simulink model "gbyk_v4b (2)"  (R2015a)
settings: Solver=ode4  SolverMode=MultiTasking  StartTime=0.0  StopTime=inf  FixedStep=BKIN_STEP_TIME  RelTol=1e-3
StartFcn:
  |  warndlg('Dexterit-E models cannot run under simulation. Please compile your model and run it from within Dexterit-E.');set_param(bdroot,'SimulationCommand','stop')
model workspace (MAT data in the model file):
  BKIN_STEP_TIME = 0.00025
  col_x = 1
  col_y = 2
  INIT_COLOR = 5
  DELAY_POST_TRIAL = 8
  BKIN_KINEMATIC_FRAME_SIZE = 400
  HIT_COLOR = 6
  E_NO_EVENT = 0
  START_TARGET_COL = 1
  MAX_REACH_TIME_COL = 7
  K_DELAY_FIXED = 3
  K_DELAY_RAND = 4
  K_TRIGGER_VEL = 5
  K_TRIGGER_POS = 6
  K_THRESH_VELMAX = 7
  E_NEW_TRIAL = 1
  E_STAY_START = 2
  E_TARGET_TRIGGER = 5
  E_HIT_TARGET = 10
  E_MISS_TARGET = 11
  K_REWARD_VAL = 1
  VISUAL_RADIUS = 3
  LOGICAL_RADIUS = 4
  STROKE_WIDTH = 7
  TEXT_COLOR = 8
  LABEL_HEIGHT = 10
  E_TOO_SLOW = 20
  K_SCORETEXT_ROW = 2
  LABEL = 9
  E_TARGETS_ON = 3
  DISPLAY_TRIAL_COL = 9
  E_SHOW_INSTRUCT = 25
  E_SHOW_SCORE = 26
  INSTRUCT_PAUSE_BTN = 2
  LABELONLY_X = 11
  LABELONLY_Y = 12
  K_PRE_REWARD_DELAY = 8
  CORR_TGT = 2
  INCORR_TGT = 3
  TGT_C_RWD_FRAC = 6
  BOX_HEIGHT = 13
  B1 = 10
  B2 = 11
  RWD_TARGETC1_COL = 4
  RWD_TARGETC2_COL = 5
undefined symbols (not defined in the file): slselsubs
libraries: Video x7, slrtlib x6, General x3, KINARM_general x3, simulink x1, xpcnilib x1
(part 2 of 2)

== stateflow chart gbyk_v4b (2)/Trial_Control ==
  settings: sampleTime=0.001
  state Initialize/
    // Both the targets and data logging are initially off.
    targetA_state = 0;
    targetB_state[1] = 0;
    targetB_state[2] = 0;
    targetC_state[1] = 0;
    targetC_state[2] = 0;
    targetC_row[1] = 10;
    targetC_row[2] = 11;
    boxState = 0;
    boxRow = 8;
    logging_enable = 0;
    score = 0;
    reward = 0;
    doreward = 0;
    feedback_text = 0;
    repeat_trial_flag = 0;
    setup_trial_flag = false;
  state MainTrial
    state ShowStartTarget/
      // Turn on first target, enable data logging, and wait for a specified time or until the hand is in the target.
      targetA_row = Trial_Protocol[START_TARGET_COL];
      targetA_state = 1;
      logging_enable = 1;
      veltrig = 0;
      postrig = 0;
      disttrig = 0;
      vmaxhit = 0;
      targetB_state[1] = 0;
      targetB_state[2] = 0;
      targetC_state[1] = 0;
      targetC_state[2] = 0;
      boxState = 0;
      tone = 0;
      reward = 0;
    state SetupTgtB/
      //if turning the targets on the for the first time (each trial), set them up. We can only do this once per trial or it will throw the counters off.
      targetB_row[1] = Trial_Protocol[B1];
      targetB_row[2] = Trial_Protocol[B2];
      corrTgt = Trial_Protocol[CORR_TGT] ;
      incorrTgt = Trial_Protocol[INCORR_TGT];
      offeredRewards[1] = Trial_Protocol[RWD_TARGETC1_COL]*Trial_Protocol[TGT_C_RWD_FRAC];
      offeredRewards[2] = Trial_Protocol[RWD_TARGETC2_COL]*Trial_Protocol[TGT_C_RWD_FRAC];
      offeredRewardsC[1] = Trial_Protocol[RWD_TARGETC1_COL];
      offeredRewardsC[2] = Trial_Protocol[RWD_TARGETC2_COL];
      setup_trial_flag = true;
    state StayAtFirstTarget/
      // Log an event that target was reached and wait for a specified time.
      // The wait time may have both a fixed and a random component. The hand must stay in the target for the full wait time.
      event_code = E_STAY_START;
      targetA_state = 1;
      tickCount = TaskwideParams[K_PRE_REWARD_DELAY];
      //TODO ask aaron if we want to show the second row values too or show nothing or just what to show before the trial starts
    state ShowAllTargets/
      // Log an event that target was reached and wait for a specified time.
      // The wait time may have both a fixed and a random component. The hand must stay in the target for the full wait time.
      event_code = E_STAY_START;
      //targetA_state = 1;
      tickCount = TaskwideParams[K_DELAY_FIXED] + TaskwideParams[K_DELAY_RAND] * rand() / RAND_MAX;
      //Show targets before the go tone - allows for comparison
      targetB_state[1] = 1;
      targetB_state[2] = 1;
      targetC_state[1] = 1;
      targetC_state[2] = 1;
      boxState = 1;
    state ShowReachTargets/
      // Turn on all reach targets and log an event indicating this has occurred. Then wait until the hand is the target or until a specified time has elapsed.
      event_code = E_TARGETS_ON;
      tickCount = Trial_Protocol[MAX_REACH_TIME_COL];
      tone = 1;
      during:
      //handvel2d = sqrt((HandVel[1])^2 + (HandVel[2])^2);
      veltrig =  (HandVel > TaskwideParams[K_TRIGGER_VEL]);
      postrig = abs(HandTgtDistance[targetA_row]) > TaskwideParams[K_TRIGGER_POS]; //TODO change this to be !box trig
      boxtrig = HandInBox[boxRow] == 1;
    state TriggerTargetC/
      // TODO event_code = E_BOX_TRIGGER;
      targetB_state[1] = 0;
      targetB_state[2] = 0;
      tone = 0;
    state TriggerTargetB/
      // if they have chosen to go for the box
      //event_code = E_CHOSE_ROW_B
      targetC_state[1] = 0;
      targetC_state[2] = 0;
      boxState = 0;
      tone = 0
      tgtdist = ( (TargetTable[targetB_row[corrTgt]][col_x] - TargetTable[targetA_row][col_x])^2.0 + (TargetTable[targetB_row[corrTgt]][col_y] - TargetTable[targetA_row][col_y])^2.0 )^0.5;
      during:
      postrig = HandInTarget[targetB_row[corrTgt]]==1;
      tgt2trig = HandInTarget[targetB_row[incorrTgt]] ==1;
      disttrigy = (HandPos[2]) > (TargetTable[targetB_row[corrTgt]][col_y])*0.01;
      disttrig = abs(HandTgtDistance[targetA_row]) > (tgtdist)*0.01;
      disttrig = disttrig && ( (TargetTable[targetB_row[corrTgt]][col_y] != TargetTable[targetA_row][col_y]) && disttrigy);
      vmaxhit = (vmaxhit || (HandVel > TaskwideParams[K_THRESH_VELMAX]));  //(sqrt(HandVel[1]^2 + HandVel[2]^2)
    state RevealCorrectTgtC/
      //event_code = E_CHOSE_TGT_C
      targetC_state[corrTgt] = 1;
      targetC_state[incorrTgt] = 0;
      during:
      //TODO fix this below
      disttrigy = (HandPos[2]) > (TargetTable[targetC_row[corrTgt]][col_y])+1;
      disttrig = abs(HandTgtDistance[targetA_row]) > (tgtdist)*0.01;
      disttrig = disttrig && disttrigy;
      postrig = HandInTarget[targetC_row[corrTgt]] ==1;
      vmaxhit = (vmaxhit || (HandVel > TaskwideParams[K_THRESH_VELMAX]));
    state TooSlowC/
      // Log a bad trial
      //event_code = E_TOO_SLOW;
      targetC_state[1] = 0;
      targetC_state[2] = 0;
      boxState = 0;
      repeat_trial_flag = 1;
      reward = 0;
      doreward = 0;
      feedback_text = -1;
      tone = 2
      tickCount = 500;
    state HitTargetC/
      // Log a successful hit
      //event_code = E_HIT_TARGETC;
      targetC_state[corrTgt] = 3;
      targetC_state[incorrTgt] = 0;
      doreward = 1;
      reward = offeredRewardsC[1];
      score += reward;
      tone = 3;
      boxState = 0
      tickCount = 500;
    state MissTargetC/
      // Log a target miss
      //event_code = E_MISS_TARGETC;
      targetC_state[1] = 0;
      targetC_state[2] = 0;
      boxState =0;
      tone = 2;
      reward = 0;
      doreward = 0;
      tickCount = 500;
    state HitTargetB/
      // Log a successful hit
      //event_code = E_HIT_TARGETB;
      targetB_state[corrTgt] = 3;
      targetB_state[incorrTgt] = 0;
      doreward = 1;
      reward = offeredRewards[1];
      score += reward;
      tone = 3;
      tickCount = 500;
    state MissTargetB/
      // Log a target miss
      //event_code = E_MISS_TARGETB;
      targetB_state[1] = 0;
      targetB_state[2] = 0;
      reward = 0;
      doreward = 0;
      tone = 2;
      tickCount = 500;
    state TooSlow/
      // Log a bad trial
      event_code = E_TOO_SLOW;
      targetB_state[1] = 0;
      targetB_state[2] = 0;
      targetC_state[1] = 0;
      targetC_state[2] = 0;
      boxState = 0;
      repeat_trial_flag = 1;
      reward = 0;
      doreward = 0;
      feedback_text = -1;
      tone = 2
      tickCount = 500;
    state EndOfTrial/
      // Set the post-trial delay.
      tickCount = Trial_Protocol[DELAY_POST_TRIAL];
    StayAtFirstTarget -> ShowStartTarget [order 2] : [HandInTarget[targetA_row] == 0]
    ShowStartTarget -> (junction 139)
    (junction 139) -> SetupTgtB [order 1] : [HandInTarget[targetA_row] == 1 && !setup_trial_flag]
    (junction 139) -> StayAtFirstTarget [order 2] : [HandInTarget[targetA_row] == 1 && setup_trial_flag]
    SetupTgtB -> StayAtFirstTarget
    StayAtFirstTarget -> ShowAllTargets [order 1] : after(tickCount, e_clk)
    ShowAllTargets -> ShowReachTargets : after(tickCount,e_clk)
    ShowReachTargets -> TooSlow [order 1] : after(tickCount, e_clk)/
        | feedback_text = -2;
        | //if the trial times out it is an error
    ShowReachTargets -> TriggerTargetC [order 3] : [after(1,e_clk) && veltrig && boxtrig]
    ShowReachTargets -> TriggerTargetB [order 2] : [after(1,e_clk) && veltrig && postrig && !boxtrig]
        | //when the hand velocity pr position exceeds the threshold
        | //shut off the second target
    TriggerTargetC -> RevealCorrectTgtC : after(1,e_clk)
    RevealCorrectTgtC -> TooSlowC [order 1] : [(after(1,e_clk) && (disttrig || postrig) && vmaxhit == 0) || after(tickCount, e_clk)]
        | //check if missed the target but moved fast enough
    RevealCorrectTgtC -> MissTargetC [order 3] : [after(1,e_clk) && (disttrig && !postrig) && vmaxhit]/
        | //check if missed the target but moved fast enough
    RevealCorrectTgtC -> HitTargetC [order 2] : [after(1,e_clk) && postrig && vmaxhit]
        | //check if hit the target and moved fast enough
    TriggerTargetB -> HitTargetB [order 3] : [after(1,e_clk) && postrig && vmaxhit]
        | //check if hit the target and moved fast enough
    TriggerTargetB -> MissTargetB [order 2] : [after(1,e_clk) && (tgt2trig || (disttrig && !postrig)) && vmaxhit]/
        | //check if missed the target but moved fast enough
    TriggerTargetB -> TooSlow [order 1] : [(after(1,e_clk) && (disttrig || postrig) && vmaxhit == 0) || after(tickCount, e_clk)]/
        | feedback_text = -1;
        | //check if missed the target but moved fast enough
    TooSlowC -> EndOfTrial
    MissTargetC -> EndOfTrial
    HitTargetC -> EndOfTrial
    HitTargetB -> EndOfTrial : after(tickCount, e_clk)
    MissTargetB -> EndOfTrial : after(tickCount, e_clk)
    TooSlow -> EndOfTrial : after(tickCount, e_clk)
  state EndInstructPause/
    instruct_num = 0;
    tickCount = Trial_Protocol[DELAY_POST_TRIAL];
    logging_enable = 1;
    score = 0;
  state Ending/
    //end the special "show score" state
    //score = 0;
    e_Trial_End;
  state ReturnToStart1/
    targetA_state=1;
    targetB_state[1] = 0;
    targetB_state[2] = 0;
    targetC_state[1] = 0;
    targetC_state[2] = 0;
    boxState = 0;
    feedback_text = 0;
    doreward = 0;
    repeat_trial_flag = 0;
    logging_enable = 1;
    setup_trial_flag = false;
  state InstructWaitState/
    //"pause" here until the button has been clicked
  state ShowScoreState/
    event_code = E_SHOW_SCORE;
    targetA_state = 0;
    targetB_state[1] = 0;
    targetB_state[2] = 0;
    targetC_state[1] = 0;
    targetC_state[2] = 0;
    boxState = 0;
    doreward = 2;
    tickCount = Trial_Protocol[MAX_REACH_TIME_COL];
    logging_enable = 0;
  state ShowInstructState/
    event_code = E_SHOW_INSTRUCT;
    targetA_state = 0;
    targetB_state[1] = 0;
    targetB_state[2] = 0;
    targetC_state[1] = 0;
    targetC_state[2] = 0;
    boxState = 0;
    doreward = 0;
    instruct_num = Trial_Protocol[DISPLAY_TRIAL_COL];
    tickCount = Trial_Protocol[MAX_REACH_TIME_COL];
    logging_enable = 0;
  state Inter_Trial_State/
    // Turn off both targets, turn off data logging, reset the
    // event code, and send the e_Trial_End Stateflow event.
    event_code = 0;
    targetA_state = 1;
    targetB_state[1] = 0;
    targetB_state[2] = 0;
    targetC_state[1] = 0;
    targetC_state[2] = 0;
    boxState = 0;
    offeredRewards[1] = 0;
    offeredRewards[2] = 0;
    feedback_text = 0;
    doreward = 0;
    setup_trial_flag = false;
    e_Trial_End;
  (default) -> Initialize
  Initialize -> ShowStartTarget [order 1] : [Trial_Protocol[DISPLAY_TRIAL_COL] == 0]
  ReturnToStart1 -> ShowStartTarget : after(1, e_clk)/
  Initialize -> ShowInstructState [order 2] : [Trial_Protocol[DISPLAY_TRIAL_COL] > 0]
      | //in case we start with an instruction trial
  Ending -> (junction 91) : after(1,e_clk)
  (junction 91) -> EndInstructPause [order 1] : [Trial_Protocol[DISPLAY_TRIAL_COL] == 0]/
      | //continue if a regular trial comes after!
  (junction 91) -> ShowInstructState [order 2] : //so we can show the score and then show instructions
      | [Trial_Protocol[DISPLAY_TRIAL_COL] > 0]
  EndInstructPause -> ReturnToStart1 : after(tickCount,e_clk)
  InstructWaitState -> Ending : e_cntl_btn/
      | event_code = 22;
  ShowScoreState -> Ending : after(tickCount,e_clk)
  ShowInstructState -> InstructWaitState : after(tickCount,e_clk)
  (junction 86) -> ReturnToStart1 [order 3] : [Trial_Protocol[DISPLAY_TRIAL_COL] == 0]
  (junction 86) -> ShowScoreState [order 1] : [Trial_Protocol[DISPLAY_TRIAL_COL] == -1]
  (junction 86) -> ShowInstructState [order 2] : [Trial_Protocol[DISPLAY_TRIAL_COL] > 0]
  Inter_Trial_State -> (junction 86) : after(1,e_clk)
  MainTrial -> Inter_Trial_State : e_ExitTrialNow/
      | tickCount = 1;
  EndOfTrial -> Inter_Trial_State : after(tickCount,e_clk)
  data: rwd_val function_output double; TgtRwdRatio function_input double; RwdVal function_input double; FixedRwdRatios1 function_input double; FixedRwdRatios2 function_input double; FixedRwdRatios3 function_input double; tIterations function_input double size=[60, 2]; TPindex function_input double; T1 function_output double; Targ1 function_input double; Targ2 function_input double; Targ1Prob function_input double; NTReps function_input double; T2 function_output double; Targ1Rwd function_input double; Targ2Rwd function_input double; RwdT1 function_output double; RwdT2 function_output double; PT1 function_output double; PT2 function_output double; tIter function_output double size=[60, 2]; r function_input double; logging_enable output double size=[2]; Trial_Protocol input double size=50; TaskwideParams input double; TrialReps input double; CurTPindex input; TargetTable input double; HandInTarget input double; event_code output uint16 [0..] =0; postrig output boolean; veltrig output boolean; disttrig output boolean; vmaxhit output boolean; targetA_row output [1..32]; targetA_state output double; targetB_row output double size=[2]; targetB_state output double size=[2]; offeredRewards output double size=2; score output double; tickCount local double; RAND_MAX constant double =32767; HandTgtDistance input double; HandPos input double; HandVel input double; doreward output double; feedback_text output int32; reward output double; instruct_num output double; tone output double; repeat_trial_flag output double; tgtdist local double; trialIterations output double size=[60, 2] =0; targetC_row output double size=[2]; targetC_state output double size=[2]; offeredRewardsC output double size=[2]; boxRow output double size=1; rwdTgts local double size=2; pTgts local double size=2; setup_trial_flag local boolean; disttrigy local boolean; tgt2trig local double; boxState output double size=1; corrTgt local double; incorrTgt local double; boxtrig local double; HandInBox input double
  data targetA_row settings: description=index of the row currently being used in the TargetTable
  events: e_clk input RISING_EDGE_EVENT; e_ExitTrialNow input EITHER_EDGE_EVENT; e_Trial_End output EITHER_EDGE_EVENT; e_cntl_btn input EITHER_EDGE_EVENT
  function rwd_val = CalcRwd(TgtRwdRatio,RwdVal,FixedRwdRatios1,FixedRwdRatios2,FixedRwdRatios3):
    | function rwd_val = CalcRwd(TgtRwdRatio,RwdVal,FixedRwdRatios1,FixedRwdRatios2,FixedRwdRatios3)
    |  
    | if TgtRwdRatio < -2
    |     rwd_val = RwdVal * FixedRwdRatios3;
    | elseif TgtRwdRatio < -1
    |     rwd_val = RwdVal * FixedRwdRatios2;
    | elseif TgtRwdRatio < 0
    |     rwd_val = RwdVal * FixedRwdRatios1;
    | else %(TgtRwdRatio > 0)
    |     rwd_val = abs(TgtRwdRatio) * RwdVal;
    | end
  function [T1,T2,RwdT1,RwdT2,PT1,PT2,tIter] = SetTargB(tIterations,TPindex,Targ1,Targ2,Targ1Prob,NTReps,Targ1Rwd,Targ2Rwd,r):
    | function [T1,T2,RwdT1,RwdT2,PT1,PT2,tIter] = SetTargB(tIterations,TPindex,Targ1,Targ2,Targ1Prob,NTReps,Targ1Rwd,Targ2Rwd,r)
    | 
    | %trialIterations is a matrix where each row corresponds to a T1TargProb, and
    | %each column counts the number of T1 and T2 iterations previously run.
    | 
    | %index the counter based on probability - but this is wrong because we can
    | %  have multiple unique trials with the same probability. So we need to
    | %  index by TP number instead!
    | %
    | % if abs(Targ1Prob - 0.5) < 1e-5
    | %     i1 = 1;
    | % elseif abs(Targ1Prob - 0.6) < 1e-5
    | %     i1 = 2;
    | % elseif abs(Targ1Prob - 0.7) < 1e-5
    | %     i1 = 3;
    | % elseif abs(Targ1Prob - 0.8) < 1e-5
    | %     i1 = 4;
    | % elseif abs(Targ1Prob - 0.9) < 1e-5
    | %     i1 = 5;
    | % elseif abs(Targ1Prob - 0.1) < 1e-5
    | %     i1 = 6;
    | % elseif abs(Targ1Prob - 0.2) < 1e-5
    | %     i1 = 7;
    | % elseif abs(Targ1Prob - 0.3) < 1e-5
    | %     i1 = 8;
    | % elseif abs(Targ1Prob - 0.4) < 1e-5
    | %     i1 = 9;
    | % elseif abs(Targ1Prob - 0.51) < 1e-5
    | %     i1 = 10;    
    | % end
    | % 
    | % Targ1Prob = round(Targ1Prob*10)/10;
    | % if abs(Targ1Prob - 0.5) < 1e-5
    | %     i1 = 1;
    | % elseif abs(Targ1Prob - 0.625) < 1e-5
    | %     i1 = 2;
    | % elseif abs(Targ1Prob - 0.75) < 1e-5
    | %     i1 = 3;
    | % elseif abs(Targ1Prob - 0.875) < 1e-5
    | %     i1 = 4;
    | % elseif abs(Targ1Prob - 0.125) < 1e-5
    | %     i1 = 5;
    | % elseif abs(Targ1Prob - 0.25) < 1e-5
    | %     i1 = 6;
    | % elseif abs(Targ1Prob - 0.375) < 1e-5
    | %     i1 = 7;
    | % elseif abs(Targ1Prob - 1.500) < 1e-5
    | %     Targ1Prob = Targ1Prob-1; %1.5 is a placeholder so we can have 2 copies of the .5 condition
    | %     i1 = 8;
    | % end
    | 
    | i1 = TPindex; %index into the trial-counter array
    | 
    | if abs(Targ1Prob - 1.500) < 1e-5
    |     Targ1Prob = Targ1Prob-1; %1.5 is a placeholder so we can have 2 copies of the .5 condition
    | end
    | Targ1Prob = round(Targ1Prob*1000)/1000; %clean up the probability value
    | 
    | 
    | %generate a random number
    | %if the random number is less than the T1 probability, set T1 to be the correct
    | %target; otherwise set T2 to be the correct target.
    | %if rand <= Targ1Prob
    | if r <= Targ1Prob
    |     tIterations(i1,1) = tIterations(i1,1)+1;
    |     if tIterations(i1,1) > NTReps*Targ1Prob %too many reps, do the other option
    |         tIterations(i1,1) = tIterations(i1,1)-1;
    |         tIterations(i1,2) = tIterations(i1,2)+1;
    |         
    |         T1 = Targ2; %swap T1 and T2
    |         T2 = Targ1;
    |         RwdT1 = Targ2Rwd;
    |         RwdT2 = Targ1Rwd;
    |         PT1 = 1-Targ1Prob;
    |         PT2 = Targ1Prob;
    |         
    |     else %T1 is good, so keep it as T1
    |         T1 = Targ1;
    |         T2 = Targ2;
    |         RwdT1 = Targ1Rwd;
    |         RwdT2 = Targ2Rwd;
    |         PT1 = Targ1Prob;
    |         PT2 = 1-Targ1Prob;
    |         
    |     end
    | else
    |     tIterations(i1,2) = tIterations(i1,2)+1;
    |     if tIterations(i1,2) > NTReps*(1-Targ1Prob) %too many reps, do the other option
    |         tIterations(i1,2) = tIterations(i1,2)-1;
    |         tIterations(i1,1) = tIterations(i1,1)+1;
    |         
    |         T1 = Targ1; %Use T1
    |         T2 = Targ2;
    |         RwdT1 = Targ1Rwd;
    |         RwdT2 = Targ2Rwd;
    |         PT1 = Targ1Prob;
    |         PT2 = 1-Targ1Prob;
    | 
    |     else
    |         
    |         T1 = Targ2; %we should be doing T2, so swap them
    |         T2 = Targ1;
    |         RwdT1 = Targ2Rwd;
    |         RwdT2 = Targ1Rwd;
    |         PT1 = 1-Targ1Prob;
    |         PT2 = Targ1Prob;
    |         
    |     end
    | end
    | 
    | tIter = tIterations; %update the trial counter and output it back to the state machine

== matlab function gbyk_v4b (2)/AddTxt2TgtB ==
  data: VCODE input; VCODE_MOD output; rewards input
function VCODE_MOD  = rwd_tgt(VCODE,rewards)
%#codegen

VCODE_MOD = VCODE;

%rewards = rwd_multipliers*rwd_val;

for a = 1:length(rewards)

    if any(rewards)>0
        jj = 1;
        label = rewards(a);
        
        if (label < 10)
            VCODE_MOD(a, jj + 14) = int32(label+int32('0'));
            
        elseif (label < 100) %score < $1
            n1 = int32(floor(double(label)/10));  %we need to cast score to a double otherwise the arithmetic is wrong!
            n2 = label - n1*10;
        
            VCODE_MOD(a, jj + 14) = int32(n1+int32('0'));
            jj = jj+1;
            VCODE_MOD(a, jj + 14) = int32(n2+int32('0'));
        else %label < 1000
            n1 = int32(floor(double(label)/100));  %we need to cast score to a double otherwise the arithmetic is wrong!
            n2 = label - n1*100;
            n2 = int32(floor(double(n2)/100));  %we need to cast score to a double otherwise the arithmetic is wrong!
            n3 = label - n1*100 - n2*10;
        
            VCODE_MOD(a, jj + 14) = int32(n1+int32('0'));
            jj = jj+1;
            VCODE_MOD(a, jj + 14) = int32(n2+int32('0'));
            jj = jj+1;
            VCODE_MOD(a, jj + 14) = int32(n3+int32('0'));
        end
        VCODE_MOD(a,jj + 1 + 14) = 0; %terminate string
    else
        VCODE_MOD(a,15) = 0; %terminate string
    end
end

== matlab function gbyk_v4b (2)/KINARM_HandInBox/Embedded MATLAB InsideTarget ==
  settings: fimath=|
      | fimath(...
      | 'RoundMode', 'floor',...
      | 'OverflowMode', 'wrap',...
      | 'ProductMode', 'KeepLSB', 'ProductWordLength', 32,...
      | 'SumMode', 'KeepLSB', 'SumWordLength', 32,...
      | 'CastBeforeSum', false)
  data: handpos input size=2; target_type input; attribcol input; num_targets input; intarget output; Target_Table input
function intarget = FIsInsideTarget(handpos, target_type, attribcol, num_targets, Target_Table)
% all dimensions in m, rad
% arguments:
% handpos: x,y positions of center of target
% attribcol: columns in target table specifying target attributes.  
% Specific to Target_Type
%	circle:
%	[X0,Y0,r...,rn] where:
%	X0,Y0 : centre of circle
%	r : logical radius of circle (i.e. radius used to determine 'in' or 'out' of target)
%	rn: logical radius of other targets (e.g. 2nd, 3rd) also specified in target row.
%   Up to 4 targets can be specified in a row
% ellipse:
%	[X0,Y0,a,b,t...,an, bn, tn] where:
%	X0,Y0 : centre of ellipse
%	a,b : major, minor radii of ellipse
%	t : rotation of ellipse in degrees
%	an,bn : major, minor radii of ellipse of other targets (e.g. 2nd, 3rd) also specified in target row
%	tn : rotation of ellipse in degrees of other targets (e.g. 2nd, 3rd) also specified in target row
%   Up to 4 targets can be specified in a row


target_col_x=1;
target_col_y=2;

x=handpos(1);
y=handpos(2);

intarget = zeros(size(Target_Table,1),5);

X0 = Target_Table(:,target_col_x)*0.01;			%Target Table sizes in cm in v1.4
Y0 = Target_Table(:,target_col_y)*0.01;			%Target Table sizes in cm in v1.4

deltax=x-X0;
deltay=y-Y0;

if target_type==1			%circle
	for target=1:num_targets
		r = Target_Table(:,attribcol(target))*0.01;			%Target Table sizes in cm in v1.4
		% simple euclidean distance
		distance2 = deltax.^2 + deltay.^2;					%distance2 is the square of the distance
	    intarget(:,target) = (distance2 <= r.^2);
	end
elseif target_type==2		%ellipse
	for target=1:num_targets
	    a = Target_Table(:,attribcol(target*3-2))*0.01;			%Target Table sizes in cm in v1.4
	    b = Target_Table(:,attribcol(target*3-1))*0.01;			%Target Table sizes in cm in v1.4	
	    t = Target_Table(:,attribcol(target*3))*(pi / 180.0);	%Target Table angles in degrees in v1.4
		sint=sin(t);
		cost=cos(t);
		xrotate=deltax.*cost+deltay.*sint;		%location of x point in ellipse's coordinate frame
		yrotate=-deltax.*sint+deltay.*cost;		%location of y point in ellipse's coordinate frame
		m=yrotate./xrotate;						%slope of line between the (x,y) to (x0,y0) in ellipse's coordinate frame
		y2sq=1./(1./(m.*a).^2+1./b.^2);			%y2sq is y2^2, where y2 is the intersection of the ellipse and the (x,y) to (x0,y0) line
	    intarget(:,target) = (yrotate.^2 <= y2sq);
    end
elseif target_type==3       %rectangle
    for target=1:num_targets
        w = Target_Table(:,attribcol(target*3-2))*0.01;  %width (sizes in cm in v1.4)
        h = Target_Table(:,attribcol(target*3-1))*0.01;  %height (sizes in cm in v1.4)
        
        if attribcol(target*3) > 0
            t = Target_Table(:,attribcol(target*3))*(pi / 180.0);  %angle (angles in degrees in v1.4)
        else
            t = zeros(size(Target_Table, 1), 1);
        end

        sint=sin(t);
        cost=cos(t);

        xrotate=deltax.*cost + deltay.*sint;   %location of x point in rectangle's coordinate frame
        yrotate=-deltax.*sint + deltay.*cost;  %location of y point in rectangle's coordinate frame

        intarget(:,target) = abs(xrotate) <= w/2 & abs(yrotate) <= h/2;
    end
elseif target_type==4       %line
    for target=1:num_targets
        % treat the line like a rectangle of height h and width w
        % determine height (stroke width) in the same fashion as in Show_Target
        if attribcol(target*3-2) == 0                     %0 column index means stroke width of 0
            h = zeros(size(Target_Table, 1), 1);
        elseif attribcol(target*3-2) < 0                  %-ve column index means stroke width of 1mm
            h = ones(size(Target_Table, 1), 1) .* 0.001;
        else
            h = Target_Table(:,attribcol(target*3-2)) * 0.01;  %target table contains width in cm
        end
        
        ex = Target_Table(:,attribcol(target*3-1))*0.01;  %endpoint in x relative to start point (cm)
        ey = Target_Table(:,attribcol(target*3))*0.01;    %endpoint in y relative to start point (cm)
        
        w = sqrt(ex.^2 + ey.^2);                          %width (cm)
        
        % determine the vector from the line's midpoint to the hand position
        handx = deltax - ex/2;
        handy = deltay - ey/2;
        
        t = atan2(ey, ex);                                %calculate angle of the line (rads)
        sint = sin(t);
        cost = cos(t);
        
        xrotate = handx.*cost + handy.*sint;   %location of x point in rectangle's coordinate frame
        yrotate = -handx.*sint + handy.*cost;  %location of y point in rectangle's coordinate frame
 
        intarget(:,target) = abs(xrotate) <= w/2 & abs(yrotate) <= h/2;
    end
elseif target_type==5  % triangle
    for target=1:num_targets
        w = Target_Table(:,attribcol(target*4-3))*0.01;         %length (sizes in cm in v1.4)
        
        % If a height column of 0 is specified, make the triangle equilateral. Otherwise, use the
        % values for height and peak offset from the target table.
        if attribcol(target*4-2) > 0
            h = Target_Table(:,attribcol(target*4-2))*0.01;  %height (sizes in cm in v1.4)
            p = Target_Table(:,attribcol(target*4-1))*0.01;  %peak offset (sizes in cm in v1.4)
        else
            h = w.*sin(pi/3.0);
            p = zeros(size(Target_Table, 1), 1);
        end
        
        if attribcol(target*4) > 0
            t = Target_Table(:,attribcol(target*4))*(pi / 180.0);  %angle (angles in degrees in v1.4)
        else
            t = zeros(size(Target_Table, 1), 1);
        end
        
        sint = sin(t);
        cost = cos(t);
        
        xrotate = deltax.*cost + deltay.*sint;   %location of x point in triangle's coordinate frame
        yrotate = -deltax.*sint + deltay.*cost;  %location of y point in triangle's coordinate frame
        
        % Perform a point-in-triangle test using Barycentric coordinates.
        A = [-w/2 - p/3, -h/3];
        B = [2*p/3, 2*h/3];
        C = [w/2 - p/3, -h/3];
        
        v0 = C - A;
        v1 = B - A;
        v2 = [xrotate, yrotate] - A;

        dot00 = v0(:,1) .* v0(:,1) + v0(:,2) .* v0(:,2);
        dot01 = v0(:,1) .* v1(:,1) + v0(:,2) .* v1(:,2);
        dot02 = v0(:,1) .* v2(:,1) + v0(:,2) .* v2(:,2);
        dot11 = v1(:,1) .* v1(:,1) + v1(:,2) .* v1(:,2);
        dot12 = v1(:,1) .* v2(:,1) + v1(:,2) .* v2(:,2);

        invDenom = 1 ./ (dot00 .* dot11 - dot01 .* dot01);
        u = (dot11 .* dot02 - dot01 .* dot12) .* invDenom;
        v = (dot00 .* dot12 - dot01 .* dot02) .* invDenom;

        intarget(:,target) = (u > 0) & (v > 0) & (u + v < 1);
    end
end

== matlab function gbyk_v4b (2)/Play Sound/Play sound over and over ==
  data: tone input; output output; beep input; errorbeep input; coin input
function output = fcn(tone,beep,errorbeep,coin)
%#codegen

persistent t last_tone_state
if isempty(t), t = 0; end
if isempty(last_tone_state), last_tone_state = 0; end

trigger = last_tone_state ~= tone;
if trigger > 0
    last_tone_state = tone;
end

output = 0;		% default
if t == 0 && trigger > 0
	% start the playing of the sound.
	t = t + 1;
end

if tone == 1
    data = beep;
elseif tone == 2
    data = errorbeep;
elseif tone == 3
    data = coin;
else 
    t = 0;
    data = 0;
end

if t > 0
	output = data(t);
	if t == length(data)
		t = 0;
	else
		t = t + 1;
	end
end

== matlab function gbyk_v4b (2)/MATLAB Function ==
  data: BlockDef input; ListReps output
function ListReps = calcListReps(BlockDef)
%#codegen

BlockDef = nonzeros(BlockDef);
%BlockDef = BlockDef(2:end);

trials = unique(BlockDef);
reps1 = sum(BlockDef == trials(1));
reps2 = sum(BlockDef == trials(2));
reps3 = sum(BlockDef == trials(3));
ListReps = round(mean([reps1,reps2,reps3]));

== matlab function gbyk_v4b (2)/DisplayText/MATLAB Function ==
  data: VCODE input; score_dbl input; VCODE_mod output; fdbk_text input
function VCODE_mod = fcn(VCODE,score_dbl,fdbk_text)


VCODE_mod = VCODE;

score = round(score_dbl);  %for display purposes, round fractional rewards

if (fdbk_text == 0)  %if this is zero, show the score
       
    
    %score is in cents. potentially need to convert to dollars
    
    if (score < 10)
        text1 = 'You earned ';
        text2 = ' cents!';
        
        textout = [text1 int2char(int32(score)) text2];
        
    elseif (score < 100) %score < $1
        text1 = 'You earned ';
        text2 = ' cents!';
        
        n1 = int32(floor(double(score)/10));  %we need to cast score to a double otherwise the arithmetic is wrong!
        n2 = score - n1*10;
        
        textout = [text1 int2char(int32(n1)) int2char(int32(n2)) text2];
        
    else %score > $1, convert to dollars to keep the score readable
        text1 = 'You earned $';
        text2 = '.';
        text3 = '!';
        
        dollars = int32(floor(double(score)/100));
        if (dollars >= 10) %double digit dollar value
            n1d = int32(floor(double(dollars)/10));
            n2d = dollars - n1d*10;
            textdollars = [int2char(int32(n1d)) int2char(int32(n2d))];
        else %single digit
            textdollars = int2char(int32(dollars));
        end
        
        cents = score-dollars*100;
        if (cents < 10)
            textcents = ['0' int2char(int32(cents))];
        else
            n1 = int32(floor(double(cents)/10));
            n2 = round(cents - n1*10);
            textcents = [int2char(int32(n1)) int2char(int32(n2))];
        end
        
        textout = [text1 textdollars text2 textcents text3];
        
    end
    
elseif (fdbk_text == 1) 
    %print "too fast"
    textout = 'Too Fast!';
    
    
elseif (fdbk_text == 2) 
    %print "too fast"
    textout = 'Too Early!';

elseif (fdbk_text == -1) 
    %print "too slow"
    
    textout = 'Too Slow!';

elseif (fdbk_text == -2) 
    %print "too fast"
    textout = 'Too Late!';


else
    textout = '';
    
end
    

%the first character is VCODE(15)
%need to translate text into ascii:
textnum = double(textout); %this quickly casts each char into a number

%make sure we won't overflow the VCODE: no more than 50 chars! we will
%clip off anything that overflows.
VCODE_mod(1,15:min([15+length(textout),64])) = textnum(1:min([length(textnum),50])); %write out as many the characters as possible into the VCODE
VCODE_mod(1,min([15+length(textout)+1,64])) = 0;  %terminate the string!



function s = int2char(n)

n = mod(n,10); %make sure we only have 1 digit or we will get a weird character!

s = char(n+int32('0')); %// add the character

== matlab function gbyk_v4b (2)/AddTxt2TgtC ==
  data: VCODE input; VCODE_MOD output; rewards input
function VCODE_MOD  = rwd_tgt(VCODE,rewards)
%#codegen

VCODE_MOD = VCODE;

%rewards = rwd_multipliers*rwd_val;

for a = 1:length(rewards)

    if any(rewards)>0
        jj = 1;
        label = rewards(a);
        
        if (label < 10)
            VCODE_MOD(a, jj + 14) = int32(label+int32('0'));
            
        elseif (label < 100) %score < $1
            n1 = int32(floor(double(label)/10));  %we need to cast score to a double otherwise the arithmetic is wrong!
            n2 = label - n1*10;
        
            VCODE_MOD(a, jj + 14) = int32(n1+int32('0'));
            jj = jj+1;
            VCODE_MOD(a, jj + 14) = int32(n2+int32('0'));
        else %label < 100
            n1 = int32(floor(double(label)/100));  %we need to cast score to a double otherwise the arithmetic is wrong!
            n2 = label - n1*100;
            n2 = int32(floor(double(n2)/100));  %we need to cast score to a double otherwise the arithmetic is wrong!
            n3 = label - n1*100 - n2*10;
        
            VCODE_MOD(a, jj + 14) = int32(n1+int32('0'));
            jj = jj+1;
            VCODE_MOD(a, jj + 14) = int32(n2+int32('0'));
            jj = jj+1;
            VCODE_MOD(a, jj + 14) = int32(n3+int32('0'));
        end
        VCODE_MOD(a,jj + 1 + 14) = 0; %terminate string
    else
        VCODE_MOD(a,15) = 0; %terminate string
    end
end

== matlab function gbyk_v4b (2)/KINARM_HandInBox/Embedded MATLAB WhichHand ==
  settings: fimath=|
      | fimath(...
      | 'RoundMode', 'floor',...
      | 'OverflowMode', 'wrap',...
      | 'ProductMode', 'KeepLSB', 'ProductWordLength', 32,...
      | 'SumMode', 'KeepLSB', 'SumWordLength', 32,...
      | 'CastBeforeSum', false)
  data: use_dominant_hand input; dominant_hand input; hand output
function hand = WhichHand(use_dominant_hand, dominant_hand)

if use_dominant_hand==1				%use the dominant hand
	hand=dominant_hand;		
else
	hand=3-dominant_hand;			%use the non-dominant hand. i.e. if dominant_hand=2, hand=1 and vice-versa
end
